simulink model "PV_array_MPPT"  (R2018a)
settings: Solver=VariableStepDiscrete  StartTime=0.0  StopTime=1  RelTol=1e-3
libraries: powerlib x10, simulink x2, pePwmGenerator x1, re_lib x1, powerlib_meascontrol x1
settings Model: Creator=apple  LastModifiedBy=apple

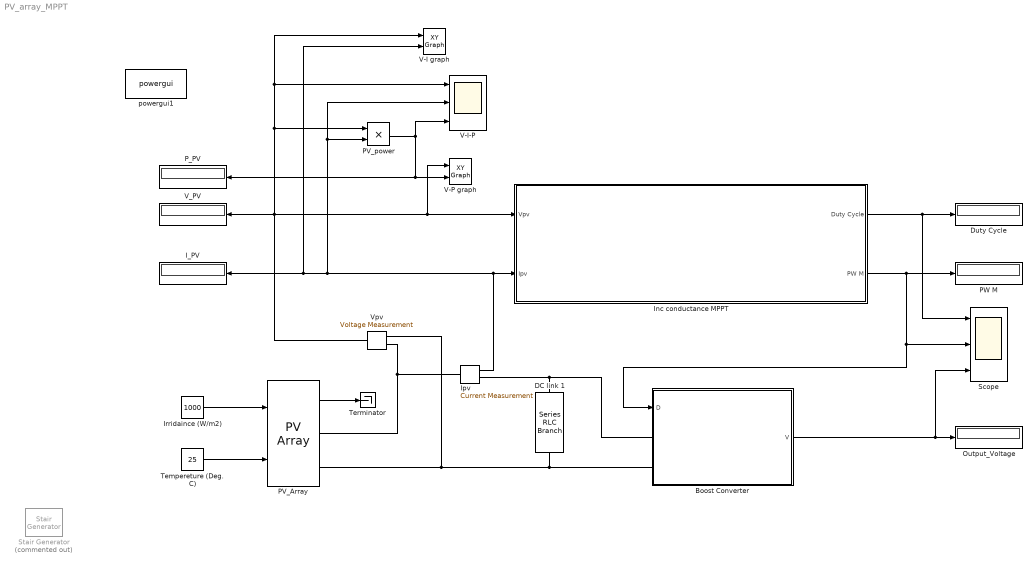
== system PV_array_MPPT ==
  Boost Converter : Subsystem
  DC link 1 : powerlib/Elements/Series RLC Branch  LConnTagsString=__new0  RConnTagsString=__new0  BranchType=C  Resistance=1  Inductance=1e-3  SetiL0=off  InitialCurrent=0  Capacitance=3e-3  Setx0=off  InitialVoltage=0  Measurements=None
  Duty Cycle : Display
  I_PV : Display
  Inc conductance MPPT : Subsystem
  Ipv : powerlib/Measurements/Current Measurement  PhasorSimulation=off  OutputType=Complex  PSBequivalent=0
  Irridaince (W/m2) : Constant  Value=1000  VectorParams1D=off
  Output_Voltage : Display
  PV_Array : re_lib/Solar/PV Array  Npar=1  Nser=1  PlotType=array @ 1000 W/m2 & specified temperatures  S_vec=[ 500 ]  Temp_C_vec=[ 25 ]  ModuleName=Aavid Solar ASMS-180M  PlotWhenSelected=off  Pm=180  Ncell=72  Voc=45  Isc=5.5  Vm=36  Im=5  beta_Voc_pc=-0.36491  alpha_Isc_pc=0.038982  beta_Voc=-0.16421  alpha_Isc=0.002144  IL=5.5239  I0=2.1103e-10  nI=1.0163  Rsh=160.0579  Rs=0.69467  BAL=off  Tc=1e-6  Tfilter=5e-5
  PV_power : Product
  PW M : Display
  P_PV : Display
  Scope : Scope  NumInputPorts=3
  Stair Generator : powerlib_meascontrol/Pulse & Signal Generators/Stair Generator  Commented=on  t=[0.2, 0.4, 0.6, 0.8, 1, 1.2, 1.4, 1.6, 1.8, 2, 2.2, 2.4, 2.6, 2.8, 3, 3.2, 3.4, 3.6, 3.8, 4, 4.2, 4.4, 4.6, 4.8]  e=[300, 400, 600, 750, 900, 1000, 900, 1000, 1100, 1200, 1000, 950, 1000, 900, 850, 850, 750, 700, 650, 600, 500, 450, 300, 200]  Ts=0.0001
      settings: SourceProductName=Simscape Power Systems
  Tempereture (Deg. C) : Constant  Value=25
  Terminator : Terminator
  "V-I graph " : simulink/Sinks/XY Graph  xmin=0  xmax=45  ymin=0  ymax=6  st=0.0001
  V-I-P : Scope  NumInputPorts=3
  V-P graph : simulink/Sinks/XY Graph  xmin=0  xmax=45  ymin=0  ymax=200  st=0.001
  V_PV : Display
  Vpv : powerlib/Measurements/Voltage Measurement  PhasorSimulation=off  OutputType=Complex  PSBequivalent=0
  powergui1 : powerlib/powergui  Priority=1  SimulationMode=Discrete  SampleTime=5e-6  frequency=60  Iterations=50  frequencyindice=0  Pbase=100e6  ErrMax=1e-4  UnitsV=kV  UnitsW=MW  buscounter=0  FunctionMessages=off  echomessages=off  EnableUseOfTLC=off  CurrentSourceSwitches=off  DisableSnubberDevices=off  DisableRonSwitches=off  DisableVfSwitches=off  DisplayEquations=off  SolverType=Tustin/Backward Euler (TBE)  Interpol=off  ExternalGateDelay=off  methode=off  Ts=100  x0status=blocks  SPID=on  SwTol=0  HookPort=off  RestoreLinks=warning  ResistiveCurrentMeasurement=off  Frange=[0:2:500]  Ylog=off  Xlog=on  ShowGrid=off  save=off  variable=ZData  structure=0  ZoomFFT=off  StartTime=0.0  cycles=1  DisplayStyle=1  fundamental=60  FreqAxis=off  MaxFrequency=1000  frequencyindicesteady=1  RmsSteady=1  display=off
  wires:
  Tempereture (Deg. C)/1 -> PV_Array/2
  PV_Array/1 -> Terminator/1
  Vpv/1 -> V-P graph/1, Inc conductance MPPT/1(Vpv), "V-I graph "/1, V-I-P/1, PV_power/1, V_PV/1
  Ipv/1 -> V-I-P/2, PV_power/2, "V-I graph "/2, I_PV/1, Inc conductance MPPT/2(Ipv)
  PV_power/1 -> V-P graph/2, P_PV/1, V-I-P/3
  Inc conductance MPPT/1(Duty Cycle) -> Duty Cycle/1, Scope/1
  Inc conductance MPPT/2(PW M) -> Boost Converter/1(D), Scope/2, PW M/1
  Boost Converter/1(V) -> Output_Voltage/1, Scope/3
  Irridaince (W/m2)/1 -> PV_Array/1
  connections:
  PV_Array/RConn1 -- Ipv/LConn1 -- Vpv/LConn1
  Boost Converter/LConn2 -- Vpv/LConn2 -- PV_Array/RConn2 -- DC link 1/RConn1
  Ipv/RConn1 -- DC link 1/LConn1 -- Boost Converter/LConn1

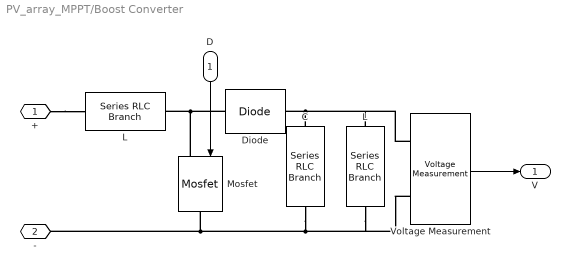
== system PV_array_MPPT/Boost Converter ==
  D : Inport
  "C " : powerlib/Elements/Series RLC Branch  LConnTagsString=__new0  RConnTagsString=__new0  BranchType=C  Resistance=1  Inductance=1e-3  SetiL0=off  InitialCurrent=0  Capacitance=100e-6  Setx0=off  InitialVoltage=0  Measurements=None
  Diode : powerlib/Power Electronics/Diode  Ron=0.001  Lon=0  Vf=0.8  IC=0  UseSnubber=0  Rs=500  Cs=250e-9  Measurements=off
  L : powerlib/Elements/Series RLC Branch  LConnTagsString=__new0  RConnTagsString=__new0  BranchType=L  Resistance=1  Inductance=100e-6  SetiL0=off  InitialCurrent=0  Capacitance=1e-6  Setx0=off  InitialVoltage=0  Measurements=None
  "L  " : powerlib/Elements/Series RLC Branch  LConnTagsString=__new0  RConnTagsString=__new0  BranchType=R  Resistance=100  Inductance=1e-3  SetiL0=off  InitialCurrent=0  Capacitance=1e-6  Setx0=off  InitialVoltage=0  Measurements=None
  Mosfet : powerlib/Power Electronics/Mosfet  Ron=0.1  Lon=0  Rd=0.01  Vfd=0  IC=0  Rs=1e5  Cs=inf  Measurements=off
  Voltage Measurement : powerlib/Measurements/Voltage Measurement  PhasorSimulation=off  OutputType=Complex  PSBequivalent=0
  + : PMIOPort  Side=Left
  - : PMIOPort  Port=2  Side=Left
  V : Outport
  wires:
  Voltage Measurement/1 -> V/1
  D/1 -> Mosfet/1
  connections:
  Mosfet/LConn1 -- L/RConn1 -- Diode/LConn1
  "C "/LConn1 -- Diode/RConn1 -- Voltage Measurement/LConn1 -- "L  "/LConn1
  +/RConn1 -- L/LConn1
  "C "/RConn1 -- "L  "/RConn1 -- Voltage Measurement/LConn2 -- Mosfet/RConn1 -- -/RConn1

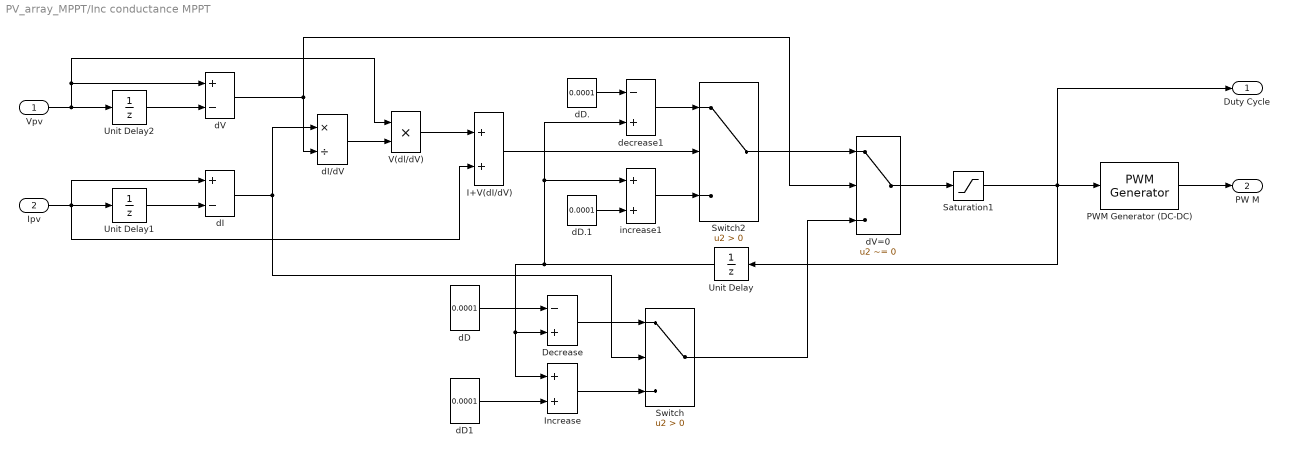
== system PV_array_MPPT/Inc conductance MPPT ==
  Vpv : Inport
  Ipv : Inport  Port=2
  Decrease : Sum  Inputs=-+
  I+V(dI/dV) : Sum
  Increase : Sum
  PWM Generator (DC-DC) : pePwmGenerator/PWM Generator  CarrCount=Up  Tper=0.001  Ts=5e-5
  Saturation1 : Saturate
  Switch : Switch  Criteria=u2 > Threshold
  Switch2 : Switch  Criteria=u2 > Threshold
  Unit Delay : UnitDelay  SampleTime=5e-6
  Unit Delay1 : UnitDelay  SampleTime=5e-5
  Unit Delay2 : UnitDelay  SampleTime=5e-5
  V(dl/dV) : Product
  dD : Constant  Value=0.0001
  dD. : Constant  Value=0.0001
  dD.1 : Constant  Value=0.0001
  dD1 : Constant  Value=0.0001
  dI : Sum  Inputs=+-
  dI/dV : Product  Inputs=*/
  dV : Sum  Inputs=+-
  dV=0 : Switch  Criteria=u2 ~= 0  Threshold=1
  decrease1 : Sum  Inputs=-+
  increase1 : Sum
  Duty Cycle : Outport
  PW M : Outport  Port=2
  wires:
  Increase/1 -> Switch/3
  decrease1/1 -> Switch2/1
  Unit Delay1/1 -> dI/2
  dD./1 -> decrease1/1
  V(dl/dV)/1 -> I+V(dI/dV)/1
  Switch2/1 -> dV=0/1
  Unit Delay2/1 -> dV/2
  I+V(dI/dV)/1 -> Switch2/2
  dI/dV/1 -> V(dl/dV)/2
  dI/1 -> Switch/2, dI/dV/1
  dD1/1 -> Increase/2
  Decrease/1 -> Switch/1
  increase1/1 -> Switch2/3
  dD/1 -> Decrease/1
  dV=0/1 -> Saturation1/1
  Vpv/1 -> V(dl/dV)/1, dV/1, Unit Delay2/1
  dD.1/1 -> increase1/2
  Ipv/1 -> I+V(dI/dV)/2, dI/1, Unit Delay1/1
  dV/1 -> dI/dV/2, dV=0/2
  PWM Generator (DC-DC)/1 -> PW M/1
  Switch/1 -> dV=0/3
  Saturation1/1 -> Duty Cycle/1, Unit Delay/1, PWM Generator (DC-DC)/1
  Unit Delay/1 -> increase1/1, decrease1/2, Decrease/2, Increase/1
